simulink model "CryoDetHcd"  (R2016b)
settings: Solver=ode45  StartTime=0.0  StopTime=1e-3  RelTol=1e-3
PreLoadFcn:
  | setup_hcd
values from neighbouring files (symbols this model uses):
  A = sqrt(0.5*erfc(x))    [setup_hcd.m]
  etaRomData = zeros(1,128)    [setup_hcd.m]
  Fadc = 614e6    (= 614000000)    [setup_hcd.m]
  freqRomData = zeros(1,128)    [setup_hcd.m]
  freqRomData1 = zeros(1,128)    [setup_hcd.m]
  freqRomData2 = zeros(1,128)    [setup_hcd.m]
  freqRomData3 = zeros(1,128)    [setup_hcd.m]
undefined symbols (not defined in the file or in its folder): AXI4, B, C, D, j, Lite
libraries: xbsIndex_r4 x2151, CryoDetLibCMB x28, hdlsllib x8, dspsigops x2, simulink x1
(part 13 of 17)

== system CryoDetHcd/DspCore/DSP/channel_processor/channel_processor_x4/128_channel_processor2/Variant Subsystem/LMS/controller/1st_harmonic2 ==
  note: D=16
  note: D=2
  note: D=5
  error : Inport
  gain : Inport  Port=2
  delay : Inport  Port=3
  enable : Inport  Port=4
  cos : Inport  Port=5
  sin : Inport  Port=6
  AddSub4 : xbsIndex_r4/AddSub  mode=Addition  use_carryin=off  use_carryout=off  en=off  latency=3  precision=User Defined  arith_type="Signed  (2's comp)"  n_bits=32  bin_pt=31  quantization=Truncate  overflow=Wrap  use_behavioral_HDL=off  hw_selection=Fabric  pipelined=off  dbl_ovrd=off  block_type=addsub
  Addressable Shift Register : xbsIndex_r4/Addressable Shift Register  infer_latency=off  depth=8  initVector=[0]  en=off  use_behavioral_HDL=off  Optimization=Resource  dbl_ovrd=off  block_type=addrsr
      settings: infoedit="Delay of configurable length.  Any element in the delay line can be addressed and driven onto the output port.<br><br>Hardware notes: Generates fast, compact FIFO-style shift registers or delay lines using SRL16/SRL32 mode of the slice LUTs"
  Addressable Shift Register1 : xbsIndex_r4/Addressable Shift Register  infer_latency=off  depth=8  initVector=[0]  en=off  use_behavioral_HDL=off  Optimization=Resource  dbl_ovrd=off  block_type=addrsr
      settings: infoedit="Delay of configurable length.  Any element in the delay line can be addressed and driven onto the output port.<br><br>Hardware notes: Generates fast, compact FIFO-style shift registers or delay lines using SRL16/SRL32 mode of the slice LUTs"
  Delay1 : xbsIndex_r4/Delay  rst=off  infoeditControl=Selection of Reset will increase slice count due to use of real FFs and instead of SRLs  en=off  latency=5  reg_retiming=off  dbl_ovrd=off  block_type=delay
  Down Sample1 : xbsIndex_r4/Down Sample  sample_ratio=128  sample_phase=First Value of Frame  en=off  rst=off  latency=0  dbl_ovrd=off  block_type=dsamp
  Down Sample2 : xbsIndex_r4/Down Sample  sample_ratio=128  sample_phase=First Value of Frame  en=off  rst=off  latency=0  dbl_ovrd=off  block_type=dsamp
  Down Sample3 : xbsIndex_r4/Down Sample  sample_ratio=128  sample_phase=First Value of Frame  en=off  rst=off  latency=0  dbl_ovrd=off  block_type=dsamp
  Mult{,1,7,13} (4 alike) : xbsIndex_r4/Mult  precision=User Defined  arith_type="Signed  (2's comp)"  n_bits=32  bin_pt=32  quantization=Truncate  overflow=Wrap  en=off  latency=3  use_behavioral_HDL=off  opt=Speed  use_embedded=on  optimum_pipeline=off  pipeline=on  dbl_ovrd=off  use_rpm=on  placement_style=Triangular  block_type=mult
  Subsystem : Subsystem
  Subsystem1 : Subsystem
  Up Sample : xbsIndex_r4/Up Sample  sample_ratio=128  copy_samples=on  en=off  latency=1  dbl_ovrd=off  block_type=usamp
  Up Sample1 : xbsIndex_r4/Up Sample  sample_ratio=128  copy_samples=on  en=off  latency=1  dbl_ovrd=off  block_type=usamp
  interleaved_accumulator1 : Subsystem
  interleaved_accumulator2 : Subsystem
  alpha1 : Outport
  alpha2 : Outport  Port=2
  Out3 : Outport  Port=3
  wires:
  error/1 -> Mult13/1, Mult7/1
  sin/1 -> Down Sample1/1, Mult/2
  cos/1 -> Down Sample2/1, Mult1/2
  Mult7/1 -> Subsystem1/2(in)
  Mult13/1 -> Subsystem/2(in)
  Mult/1 -> AddSub4/1
  Mult1/1 -> AddSub4/2
  AddSub4/1 -> Out3/1
  interleaved_accumulator2/1(Out1) -> alpha2/1, Mult1/1  "alpha2"
  interleaved_accumulator1/1(Out1) -> alpha1/1, Mult/1  "alpha1"
  Subsystem/1(out) -> interleaved_accumulator1/1(In1)
  Down Sample1/1 -> Addressable Shift Register/1
  Down Sample2/1 -> Addressable Shift Register1/1
  Addressable Shift Register1/1 -> Up Sample/1
  Addressable Shift Register/1 -> Up Sample1/1
  delay/1 -> Down Sample3/1
  Subsystem1/1(out) -> interleaved_accumulator2/1(In1)
  gain/1 -> Subsystem1/1(gain), Subsystem/1(gain)
  Down Sample3/1 -> Addressable Shift Register1/2, Addressable Shift Register/2
  Up Sample/1 -> Mult7/2
  Up Sample1/1 -> Mult13/2
  enable/1 -> Delay1/1
  Delay1/1 -> interleaved_accumulator2/2(enable), interleaved_accumulator1/2(enable)

== system CryoDetHcd/DspCore/DSP/channel_processor/channel_processor_x4/128_channel_processor2/Variant Subsystem/LMS/controller/DC ==
  error : Inport
  gain : Inport  Port=2
  dc_offset : Inport  Port=3
  enable : Inport  Port=4
  AddSub4 : xbsIndex_r4/AddSub  mode=Addition  use_carryin=off  use_carryout=off  en=off  latency=3  precision=User Defined  arith_type="Signed  (2's comp)"  n_bits=32  bin_pt=31  quantization=Truncate  overflow=Wrap  use_behavioral_HDL=off  hw_selection=Fabric  pipelined=off  dbl_ovrd=off  block_type=addsub
  Delay : xbsIndex_r4/Delay  rst=off  infoeditControl=Selection of Reset will increase slice count due to use of real FFs and instead of SRLs  en=off  latency=3  reg_retiming=off  dbl_ovrd=off  block_type=delay
  Delay1 : xbsIndex_r4/Delay  rst=off  infoeditControl=Selection of Reset will increase slice count due to use of real FFs and instead of SRLs  en=off  latency=3  reg_retiming=off  dbl_ovrd=off  block_type=delay
  Delay2 : xbsIndex_r4/Delay  rst=off  infoeditControl=Selection of Reset will increase slice count due to use of real FFs and instead of SRLs  en=off  latency=13  reg_retiming=off  dbl_ovrd=off  block_type=delay
  Delay3 : xbsIndex_r4/Delay  rst=off  infoeditControl=Selection of Reset will increase slice count due to use of real FFs and instead of SRLs  en=off  latency=5  reg_retiming=off  dbl_ovrd=off  block_type=delay
  Scope : Scope  NumInputPorts=4
  Subsystem : Subsystem
  interleaved_accumulator2 : Subsystem
  alpha1 : Outport
  Out3 : Outport  Port=2
  wires:
  gain/1 -> Subsystem/1(gain)
  Subsystem/1(out) -> Scope/2, interleaved_accumulator2/1(In1)
  interleaved_accumulator2/1(Out1) -> Scope/3, Delay1/1, alpha1/1  "alpha1"
  AddSub4/1 -> Out3/1
  error/1 -> Scope/1, Delay/1
  dc_offset/1 -> Delay2/1
  Delay/1 -> Subsystem/2(in)
  Delay1/1 -> AddSub4/1
  Delay2/1 -> AddSub4/2
  enable/1 -> Delay3/1
  Delay3/1 -> Scope/4, interleaved_accumulator2/2(enable)

== system CryoDetHcd/DspCore/DSP/channel_processor/channel_processor_x4/128_channel_processor2/Variant Subsystem/LMS/controller/freqs ==
  rst : Inport
  freq : Inport  Port=2
  AddSub : xbsIndex_r4/AddSub  mode=Addition  use_carryin=off  use_carryout=off  en=off  latency=1  precision=User Defined  arith_type=Unsigned  n_bits=16  bin_pt=16  quantization=Truncate  overflow=Wrap  use_behavioral_HDL=off  hw_selection=Fabric  pipelined=off  dbl_ovrd=off  block_type=addsub
  Addressable Shift Register : xbsIndex_r4/Addressable Shift Register  infer_latency=off  depth=128  initVector=[ 1 1 1 zeros(1,125)]  en=off  use_behavioral_HDL=off  Optimization=Resource  dbl_ovrd=off  block_type=addrsr
      settings: infoedit="Delay of configurable length.  Any element in the delay line can be addressed and driven onto the output port.<br><br>Hardware notes: Generates fast, compact FIFO-style shift registers or delay lines using SRL16/SRL32 mode of the slice LUTs"
  Addressable Shift Register1 : xbsIndex_r4/Addressable Shift Register  infer_latency=off  depth=128  initVector=[2 1 0 zeros(1,125)]  en=off  use_behavioral_HDL=off  Optimization=Resource  dbl_ovrd=off  block_type=addrsr
      settings: infoedit="Delay of configurable length.  Any element in the delay line can be addressed and driven onto the output port.<br><br>Hardware notes: Generates fast, compact FIFO-style shift registers or delay lines using SRL16/SRL32 mode of the slice LUTs"
  Assert : xbsIndex_r4/Assert  assert_type=on  type_source=Explicitly  gui_display_data_type=Boolean  arith_type=Boolean  n_bits=16  bin_pt=14  preci_type=Single  exp_width=8  frac_width=24  assert_rate=on  rate_source=Explicitly  period=2/Fadc  output_port=on  block_type=assert
  Assert1 : xbsIndex_r4/Assert  assert_type=on  type_source=Explicitly  gui_display_data_type=Fixed-point  arith_type=Unsigned  n_bits=2  bin_pt=0  preci_type=Single  exp_width=8  frac_width=24  assert_rate=on  rate_source=Explicitly  period=2/Fadc  output_port=on  block_type=assert
  Constant : xbsIndex_r4/Constant  const=126  gui_display_data_type=Fixed-point  arith_type=Unsigned  n_bits=7  bin_pt=0  preci_type=Single  exp_width=8  frac_width=24  explicit_period=off  period=1  equ=P=C  opselect=C  inp2=PCIN>>17  opr=+  inp1=P  carry=CIN  dbl_ovrd=off  block_type=constant
  Constant3 : xbsIndex_r4/Constant  const=126  gui_display_data_type=Fixed-point  arith_type=Unsigned  n_bits=7  bin_pt=0  preci_type=Single  exp_width=8  frac_width=24  explicit_period=off  period=1  equ=P=C  opselect=C  inp2=PCIN>>17  opr=+  inp1=P  carry=CIN  dbl_ovrd=off  block_type=constant
  Constant4 : xbsIndex_r4/Constant  const=1.0  gui_display_data_type=Boolean  arith_type=Boolean  n_bits=16  bin_pt=14  preci_type=Single  exp_width=8  frac_width=24  explicit_period=off  period=1  equ=P=C  opselect=C  inp2=PCIN>>17  opr=+  inp1=P  carry=CIN  dbl_ovrd=off  block_type=constant
  Constant5 : xbsIndex_r4/Constant  const=0  gui_display_data_type=Boolean  arith_type=Boolean  n_bits=16  bin_pt=14  preci_type=Single  exp_width=8  frac_width=24  explicit_period=off  period=1  equ=P=C  opselect=C  inp2=PCIN>>17  opr=+  inp1=P  carry=CIN  dbl_ovrd=off  block_type=constant
  Constant6 : xbsIndex_r4/Constant  const=0  gui_display_data_type=Fixed-point  arith_type=Unsigned  n_bits=2  bin_pt=0  preci_type=Single  exp_width=8  frac_width=24  explicit_period=off  period=1  equ=P=C  opselect=C  inp2=PCIN>>17  opr=+  inp1=P  carry=CIN  dbl_ovrd=off  block_type=constant
  Constant7 : xbsIndex_r4/Constant  const=1  gui_display_data_type=Fixed-point  arith_type=Unsigned  n_bits=2  bin_pt=0  preci_type=Single  exp_width=8  frac_width=24  explicit_period=off  period=1  equ=P=C  opselect=C  inp2=PCIN>>17  opr=+  inp1=P  carry=CIN  dbl_ovrd=off  block_type=constant
  Constant8 : xbsIndex_r4/Constant  const=2  gui_display_data_type=Fixed-point  arith_type=Unsigned  n_bits=2  bin_pt=0  preci_type=Single  exp_width=8  frac_width=24  explicit_period=off  period=1  equ=P=C  opselect=C  inp2=PCIN>>17  opr=+  inp1=P  carry=CIN  dbl_ovrd=off  block_type=constant
  "DDS Compiler 6.0 " : xbsIndex_r4/DDS Compiler 6.0   partspresent=Phase_Generator_and_SIN_COS_LUT  dds_clock_rate=38.4  channels=3  mode_of_operation=Standard  modulus=9  parameter_entry=Hardware_Parameters  spurious_free_dynamic_range=45  frequency_resolution=0.4  noise_shaping=None  phase_width=16  output_width=18  output_selection=Sine_and_Cosine  negative_sine=off  negative_cosine=off  amplitude_mode=Full_Range  memory_type=Auto  optimization_goal=Speed  dsp48_use=Minimal  resync=off  latency_configuration=Auto  latency=1  has_phase_out=off  has_aclken=off  has_aresetn=on  explicit_period=off  period=1  data_has_tlast=Not_Required  has_tready=on  s_phase_has_tuser=User_Field  m_data_has_tuser=User_Field  m_phase_has_tuser=Not_Required  s_phase_tuser_width=2  output_form=Twos_Complement  s_config_sync_mode=On_Packet  phase_increment=Streaming  output_frequency1=0  output_frequency2=0  output_frequency3=0  output_frequency4=0  output_frequency5=0  output_frequency6=0  output_frequency7=0  output_frequency8=0  output_frequency9=0  output_frequency10=0  output_frequency11=0  output_frequency12=0  output_frequency13=0  output_frequency14=0  output_frequency15=0  output_frequency16=0  pinc1='0'  pinc2='0'  pinc3='0'  pinc4='0'  pinc5='0'  pinc6='0'  pinc7='0'  pinc8='0'  pinc9='0'  pinc10='0'  pinc11='0'  pinc12='0'  pinc13='0'  pinc14='0'  pinc15='0'  pinc16='0'  phase_offset=None  phase_offset_angles1=0  phase_offset_angles2=0  phase_offset_angles3=0  phase_offset_angles4=0  phase_offset_angles5=0  phase_offset_angles6=0  phase_offset_angles7=0  phase_offset_angles8=0  phase_offset_angles9=0  phase_offset_angles10=0  phase_offset_angles11=0  phase_offset_angles12=0  phase_offset_angles13=0  phase_offset_angles14=0  phase_offset_angles15=0  phase_offset_angles16=0  poff1='0'  poff2='0'  poff3='0'  poff4='0'  poff5='0'  poff6='0'  poff7='0'  poff8='0'  poff9='0'  poff10='0'  poff11='0'  poff12='0'  poff13='0'  poff14='0'  poff15='0'  poff16='0'  trim_axipin_name=on  simulation_type=hybrid_sim  simulation_model=sysgen:xddsv6_0_cmodel  data_path_portlist={ 's_axis_config_tdata_poff', 's_axis_config_tdata_chan0_poff', 's_axis_config_tdata_pinc', 's_axis_config_tdata_chan0_pinc', 's_axis_phase_tdata_resync', 's_axis_phase_tdata_chan0_resync', 's_axis_phase_tdata_poff', 's_axis_phase_tdata_chan0_poff', 's_axis_phase_tdata_pinc', 's_axis_phase_tdata_chan0_pinc', 's_axis_phase_tdata_phase_in', 'm_axis_data_tdata_sine', 'm_axis_data_tdata_chan0_sine', 'm_axis_data_tdata_cosine', 'm_axis_data_tdata_chan0_cosine', 'm_axis_phase_tdata_phase_out', 'm_axis_phase_tdata_chan0_phase_out'}  por_mode=false  gui_behaviour=Sysgen  ip_name=DDS Compiler  ip_version=6.0  dsptool_ready=true  wrapper_available=true  port_translation_map={ 'aclken' => 'en', 'aresetn' => 'rst' }  ipcore_usecache=true  ipcore_useipmodelcache=true  ipcore_xco_need_fpga_part=true  ipcore_verbose=false  block_type=dds_compiler_v6_0
  Inverter : xbsIndex_r4/Inverter  en=off  latency=0  dbl_ovrd=off  block_type=inv
  Mux5 : xbsIndex_r4/Mux  inputs=3  en=off  latency=1  precision=Full  arith_type=Unsigned  n_bits=16  bin_pt=14  quantization=Truncate  overflow=Wrap  dbl_ovrd=off  block_type=mux
  Register{1..3,8,12..16} (9 alike) : xbsIndex_r4/Register  init=0  rst=off  en=off  dbl_ovrd=off  block_type=register
  Shift : xbsIndex_r4/Shift  shift_dir=Left  shift_bits=1  en=off  latency=1  precision=User Defined  arith_type=Unsigned  n_bits=16  bin_pt=16  quantization=Truncate  overflow=Wrap  dbl_ovrd=off  block_type=shift
  Subsystem : Subsystem
  Subsystem1 : Subsystem
  Subsystem2 : Subsystem
  Terminator : Terminator
  Terminator1 : Terminator
  Terminator2 : Terminator
  h0_0 : Outport
  h0_1 : Outport  Port=2
  h1_0 : Outport  Port=3
  h1_1 : Outport  Port=4
  h2_0 : Outport  Port=5
  h2_1 : Outport  Port=6
  wires:
  "DDS Compiler 6.0 "/7 -> Terminator2/1
  "DDS Compiler 6.0 "/1 -> Terminator/1
  "DDS Compiler 6.0 "/6 -> Terminator1/1
  Addressable Shift Register/1 -> Register8/1
  Register8/1 -> Register13/1, Assert/1
  Constant/1 -> Addressable Shift Register/2
  Addressable Shift Register1/1 -> Register12/1
  Register12/1 -> Register1/1, Mux5/1, Assert1/1
  Constant3/1 -> Addressable Shift Register1/2
  Register13/1 -> "DDS Compiler 6.0 "/1
  Register14/1 -> Shift/1, AddSub/1, Mux5/2
  Shift/1 -> AddSub/2, Mux5/3
  AddSub/1 -> Mux5/4
  Mux5/1 -> "DDS Compiler 6.0 "/2
  Constant4/1 -> "DDS Compiler 6.0 "/5
  Constant5/1 -> "DDS Compiler 6.0 "/3
  "DDS Compiler 6.0 "/2 -> Register2/1
  "DDS Compiler 6.0 "/3 -> Register15/1
  "DDS Compiler 6.0 "/4 -> Register16/1
  Register15/1 -> Subsystem/3(In3), Subsystem2/3(In3), Subsystem1/3(In3)
  Constant6/1 -> Subsystem/1(Chan)
  Constant8/1 -> Subsystem2/1(Chan)
  Constant7/1 -> Subsystem1/1(Chan)
  freq/1 -> Register14/1
  Assert/1 -> Addressable Shift Register/1
  Assert1/1 -> Addressable Shift Register1/1
  Register3/1 -> Subsystem/2(In2), Subsystem2/2(In2), Subsystem1/2(In2)
  Register2/1 -> Subsystem2/5(valid), Subsystem1/5(valid), Subsystem/5(valid)
  Register16/1 -> Subsystem1/4(In4), Subsystem/4(In4), Subsystem2/4(In4)
  rst/1 -> Inverter/1
  Inverter/1 -> "DDS Compiler 6.0 "/6
  Register1/1 -> "DDS Compiler 6.0 "/4
  "DDS Compiler 6.0 "/5 -> Register3/1
  Subsystem2/2(Out3) -> h2_1/1
  Subsystem2/1(Out2) -> h2_0/1
  Subsystem1/2(Out3) -> h1_1/1
  Subsystem1/1(Out2) -> h1_0/1
  Subsystem/2(Out3) -> h0_1/1
  Subsystem/1(Out2) -> h0_0/1

== system CryoDetHcd/DspCore/DSP/channel_processor/channel_processor_x4/128_channel_processor3/Variant Subsystem/LMS/controller/1st_harmonic ==
  note: D=5
  note: D=2
  note: D=16
  error : Inport
  gain : Inport  Port=2
  delay : Inport  Port=3
  enable : Inport  Port=4
  cos : Inport  Port=5
  sin : Inport  Port=6
  AddSub4 : xbsIndex_r4/AddSub  mode=Addition  use_carryin=off  use_carryout=off  en=off  latency=3  precision=User Defined  arith_type="Signed  (2's comp)"  n_bits=32  bin_pt=31  quantization=Truncate  overflow=Wrap  use_behavioral_HDL=off  hw_selection=Fabric  pipelined=off  dbl_ovrd=off  block_type=addsub
  Addressable Shift Register : xbsIndex_r4/Addressable Shift Register  infer_latency=off  depth=8  initVector=[0]  en=off  use_behavioral_HDL=off  Optimization=Resource  dbl_ovrd=off  block_type=addrsr
      settings: infoedit="Delay of configurable length.  Any element in the delay line can be addressed and driven onto the output port.<br><br>Hardware notes: Generates fast, compact FIFO-style shift registers or delay lines using SRL16/SRL32 mode of the slice LUTs"
  Addressable Shift Register1 : xbsIndex_r4/Addressable Shift Register  infer_latency=off  depth=8  initVector=[0]  en=off  use_behavioral_HDL=off  Optimization=Resource  dbl_ovrd=off  block_type=addrsr
      settings: infoedit="Delay of configurable length.  Any element in the delay line can be addressed and driven onto the output port.<br><br>Hardware notes: Generates fast, compact FIFO-style shift registers or delay lines using SRL16/SRL32 mode of the slice LUTs"
  Delay1 : xbsIndex_r4/Delay  rst=off  infoeditControl=Selection of Reset will increase slice count due to use of real FFs and instead of SRLs  en=off  latency=5  reg_retiming=off  dbl_ovrd=off  block_type=delay
  Down Sample1 : xbsIndex_r4/Down Sample  sample_ratio=128  sample_phase=First Value of Frame  en=off  rst=off  latency=0  dbl_ovrd=off  block_type=dsamp
  Down Sample2 : xbsIndex_r4/Down Sample  sample_ratio=128  sample_phase=First Value of Frame  en=off  rst=off  latency=0  dbl_ovrd=off  block_type=dsamp
  Down Sample3 : xbsIndex_r4/Down Sample  sample_ratio=128  sample_phase=First Value of Frame  en=off  rst=off  latency=0  dbl_ovrd=off  block_type=dsamp
  Mult{,1,7,13} (4 alike) : xbsIndex_r4/Mult  precision=User Defined  arith_type="Signed  (2's comp)"  n_bits=32  bin_pt=32  quantization=Truncate  overflow=Wrap  en=off  latency=3  use_behavioral_HDL=off  opt=Speed  use_embedded=on  optimum_pipeline=off  pipeline=on  dbl_ovrd=off  use_rpm=on  placement_style=Triangular  block_type=mult
  Subsystem : Subsystem
  Subsystem1 : Subsystem
  Up Sample : xbsIndex_r4/Up Sample  sample_ratio=128  copy_samples=on  en=off  latency=1  dbl_ovrd=off  block_type=usamp
  Up Sample1 : xbsIndex_r4/Up Sample  sample_ratio=128  copy_samples=on  en=off  latency=1  dbl_ovrd=off  block_type=usamp
  interleaved_accumulator1 : Subsystem
  interleaved_accumulator2 : Subsystem
  alpha1 : Outport
  alpha2 : Outport  Port=2
  Out3 : Outport  Port=3
  wires:
  Delay1/1 -> interleaved_accumulator1/2(enable), interleaved_accumulator2/2(enable)
  enable/1 -> Delay1/1
  Up Sample1/1 -> Mult13/2
  Up Sample/1 -> Mult7/2
  Down Sample3/1 -> Addressable Shift Register/2, Addressable Shift Register1/2
  gain/1 -> Subsystem/1(gain), Subsystem1/1(gain)
  Subsystem1/1(out) -> interleaved_accumulator2/1(In1)
  delay/1 -> Down Sample3/1
  Addressable Shift Register/1 -> Up Sample1/1
  Addressable Shift Register1/1 -> Up Sample/1
  Down Sample2/1 -> Addressable Shift Register1/1
  Down Sample1/1 -> Addressable Shift Register/1
  Subsystem/1(out) -> interleaved_accumulator1/1(In1)
  interleaved_accumulator1/1(Out1) -> Mult/1, alpha1/1  "alpha1"
  interleaved_accumulator2/1(Out1) -> Mult1/1, alpha2/1  "alpha2"
  AddSub4/1 -> Out3/1
  Mult1/1 -> AddSub4/2
  Mult/1 -> AddSub4/1
  Mult13/1 -> Subsystem/2(in)
  Mult7/1 -> Subsystem1/2(in)
  cos/1 -> Mult1/2, Down Sample2/1
  sin/1 -> Mult/2, Down Sample1/1
  error/1 -> Mult7/1, Mult13/1

== system CryoDetHcd/DspCore/DSP/channel_processor/channel_processor_x4/128_channel_processor3/Variant Subsystem/LMS/controller/1st_harmonic1 ==
  note: D=16
  note: D=2
  note: D=5
  error : Inport
  gain : Inport  Port=2
  delay : Inport  Port=3
  enable : Inport  Port=4
  cos : Inport  Port=5
  sin : Inport  Port=6
  AddSub4 : xbsIndex_r4/AddSub  mode=Addition  use_carryin=off  use_carryout=off  en=off  latency=3  precision=User Defined  arith_type="Signed  (2's comp)"  n_bits=32  bin_pt=31  quantization=Truncate  overflow=Wrap  use_behavioral_HDL=off  hw_selection=Fabric  pipelined=off  dbl_ovrd=off  block_type=addsub
  Addressable Shift Register : xbsIndex_r4/Addressable Shift Register  infer_latency=off  depth=8  initVector=[0]  en=off  use_behavioral_HDL=off  Optimization=Resource  dbl_ovrd=off  block_type=addrsr
      settings: infoedit="Delay of configurable length.  Any element in the delay line can be addressed and driven onto the output port.<br><br>Hardware notes: Generates fast, compact FIFO-style shift registers or delay lines using SRL16/SRL32 mode of the slice LUTs"
  Addressable Shift Register1 : xbsIndex_r4/Addressable Shift Register  infer_latency=off  depth=8  initVector=[0]  en=off  use_behavioral_HDL=off  Optimization=Resource  dbl_ovrd=off  block_type=addrsr
      settings: infoedit="Delay of configurable length.  Any element in the delay line can be addressed and driven onto the output port.<br><br>Hardware notes: Generates fast, compact FIFO-style shift registers or delay lines using SRL16/SRL32 mode of the slice LUTs"
  Delay1 : xbsIndex_r4/Delay  rst=off  infoeditControl=Selection of Reset will increase slice count due to use of real FFs and instead of SRLs  en=off  latency=5  reg_retiming=off  dbl_ovrd=off  block_type=delay
  Down Sample1 : xbsIndex_r4/Down Sample  sample_ratio=128  sample_phase=First Value of Frame  en=off  rst=off  latency=0  dbl_ovrd=off  block_type=dsamp
  Down Sample2 : xbsIndex_r4/Down Sample  sample_ratio=128  sample_phase=First Value of Frame  en=off  rst=off  latency=0  dbl_ovrd=off  block_type=dsamp
  Down Sample3 : xbsIndex_r4/Down Sample  sample_ratio=128  sample_phase=First Value of Frame  en=off  rst=off  latency=0  dbl_ovrd=off  block_type=dsamp
  Mult{,1,7,13} (4 alike) : xbsIndex_r4/Mult  precision=User Defined  arith_type="Signed  (2's comp)"  n_bits=32  bin_pt=32  quantization=Truncate  overflow=Wrap  en=off  latency=3  use_behavioral_HDL=off  opt=Speed  use_embedded=on  optimum_pipeline=off  pipeline=on  dbl_ovrd=off  use_rpm=on  placement_style=Triangular  block_type=mult
  Subsystem : Subsystem
  Subsystem1 : Subsystem
  Up Sample : xbsIndex_r4/Up Sample  sample_ratio=128  copy_samples=on  en=off  latency=1  dbl_ovrd=off  block_type=usamp
  Up Sample1 : xbsIndex_r4/Up Sample  sample_ratio=128  copy_samples=on  en=off  latency=1  dbl_ovrd=off  block_type=usamp
  interleaved_accumulator1 : Subsystem
  interleaved_accumulator2 : Subsystem
  alpha1 : Outport
  alpha2 : Outport  Port=2
  Out3 : Outport  Port=3
  wires:
  error/1 -> Mult13/1, Mult7/1
  sin/1 -> Down Sample1/1, Mult/2
  cos/1 -> Down Sample2/1, Mult1/2
  Mult7/1 -> Subsystem1/2(in)
  Mult13/1 -> Subsystem/2(in)
  Mult/1 -> AddSub4/1
  Mult1/1 -> AddSub4/2
  AddSub4/1 -> Out3/1
  interleaved_accumulator2/1(Out1) -> alpha2/1, Mult1/1  "alpha2"
  interleaved_accumulator1/1(Out1) -> alpha1/1, Mult/1  "alpha1"
  Subsystem/1(out) -> interleaved_accumulator1/1(In1)
  Down Sample1/1 -> Addressable Shift Register/1
  Down Sample2/1 -> Addressable Shift Register1/1
  Addressable Shift Register1/1 -> Up Sample/1
  Addressable Shift Register/1 -> Up Sample1/1
  delay/1 -> Down Sample3/1
  Subsystem1/1(out) -> interleaved_accumulator2/1(In1)
  gain/1 -> Subsystem1/1(gain), Subsystem/1(gain)
  Down Sample3/1 -> Addressable Shift Register1/2, Addressable Shift Register/2
  Up Sample/1 -> Mult7/2
  Up Sample1/1 -> Mult13/2
  enable/1 -> Delay1/1
  Delay1/1 -> interleaved_accumulator2/2(enable), interleaved_accumulator1/2(enable)

== system CryoDetHcd/DspCore/DSP/channel_processor/channel_processor_x4/128_channel_processor3/Variant Subsystem/LMS/controller/1st_harmonic2 ==
  note: D=5
  note: D=2
  note: D=16
  error : Inport
  gain : Inport  Port=2
  delay : Inport  Port=3
  enable : Inport  Port=4
  cos : Inport  Port=5
  sin : Inport  Port=6
  AddSub4 : xbsIndex_r4/AddSub  mode=Addition  use_carryin=off  use_carryout=off  en=off  latency=3  precision=User Defined  arith_type="Signed  (2's comp)"  n_bits=32  bin_pt=31  quantization=Truncate  overflow=Wrap  use_behavioral_HDL=off  hw_selection=Fabric  pipelined=off  dbl_ovrd=off  block_type=addsub
  Addressable Shift Register : xbsIndex_r4/Addressable Shift Register  infer_latency=off  depth=8  initVector=[0]  en=off  use_behavioral_HDL=off  Optimization=Resource  dbl_ovrd=off  block_type=addrsr
      settings: infoedit="Delay of configurable length.  Any element in the delay line can be addressed and driven onto the output port.<br><br>Hardware notes: Generates fast, compact FIFO-style shift registers or delay lines using SRL16/SRL32 mode of the slice LUTs"
  Addressable Shift Register1 : xbsIndex_r4/Addressable Shift Register  infer_latency=off  depth=8  initVector=[0]  en=off  use_behavioral_HDL=off  Optimization=Resource  dbl_ovrd=off  block_type=addrsr
      settings: infoedit="Delay of configurable length.  Any element in the delay line can be addressed and driven onto the output port.<br><br>Hardware notes: Generates fast, compact FIFO-style shift registers or delay lines using SRL16/SRL32 mode of the slice LUTs"
  Delay1 : xbsIndex_r4/Delay  rst=off  infoeditControl=Selection of Reset will increase slice count due to use of real FFs and instead of SRLs  en=off  latency=5  reg_retiming=off  dbl_ovrd=off  block_type=delay
  Down Sample1 : xbsIndex_r4/Down Sample  sample_ratio=128  sample_phase=First Value of Frame  en=off  rst=off  latency=0  dbl_ovrd=off  block_type=dsamp
  Down Sample2 : xbsIndex_r4/Down Sample  sample_ratio=128  sample_phase=First Value of Frame  en=off  rst=off  latency=0  dbl_ovrd=off  block_type=dsamp
  Down Sample3 : xbsIndex_r4/Down Sample  sample_ratio=128  sample_phase=First Value of Frame  en=off  rst=off  latency=0  dbl_ovrd=off  block_type=dsamp
  Mult{,1,7,13} (4 alike) : xbsIndex_r4/Mult  precision=User Defined  arith_type="Signed  (2's comp)"  n_bits=32  bin_pt=32  quantization=Truncate  overflow=Wrap  en=off  latency=3  use_behavioral_HDL=off  opt=Speed  use_embedded=on  optimum_pipeline=off  pipeline=on  dbl_ovrd=off  use_rpm=on  placement_style=Triangular  block_type=mult
  Subsystem : Subsystem
  Subsystem1 : Subsystem
  Up Sample : xbsIndex_r4/Up Sample  sample_ratio=128  copy_samples=on  en=off  latency=1  dbl_ovrd=off  block_type=usamp
  Up Sample1 : xbsIndex_r4/Up Sample  sample_ratio=128  copy_samples=on  en=off  latency=1  dbl_ovrd=off  block_type=usamp
  interleaved_accumulator1 : Subsystem
  interleaved_accumulator2 : Subsystem
  alpha1 : Outport
  alpha2 : Outport  Port=2
  Out3 : Outport  Port=3
  wires:
  Delay1/1 -> interleaved_accumulator1/2(enable), interleaved_accumulator2/2(enable)
  enable/1 -> Delay1/1
  Up Sample1/1 -> Mult13/2
  Up Sample/1 -> Mult7/2
  Down Sample3/1 -> Addressable Shift Register/2, Addressable Shift Register1/2
  gain/1 -> Subsystem/1(gain), Subsystem1/1(gain)
  Subsystem1/1(out) -> interleaved_accumulator2/1(In1)
  delay/1 -> Down Sample3/1
  Addressable Shift Register/1 -> Up Sample1/1
  Addressable Shift Register1/1 -> Up Sample/1
  Down Sample2/1 -> Addressable Shift Register1/1
  Down Sample1/1 -> Addressable Shift Register/1
  Subsystem/1(out) -> interleaved_accumulator1/1(In1)
  interleaved_accumulator1/1(Out1) -> Mult/1, alpha1/1  "alpha1"
  interleaved_accumulator2/1(Out1) -> Mult1/1, alpha2/1  "alpha2"
  AddSub4/1 -> Out3/1
  Mult1/1 -> AddSub4/2
  Mult/1 -> AddSub4/1
  Mult13/1 -> Subsystem/2(in)
  Mult7/1 -> Subsystem1/2(in)
  cos/1 -> Mult1/2, Down Sample2/1
  sin/1 -> Mult/2, Down Sample1/1
  error/1 -> Mult7/1, Mult13/1

== system CryoDetHcd/DspCore/DSP/channel_processor/channel_processor_x4/128_channel_processor3/Variant Subsystem/LMS/controller/DC ==
  error : Inport
  gain : Inport  Port=2
  dc_offset : Inport  Port=3
  enable : Inport  Port=4
  AddSub4 : xbsIndex_r4/AddSub  mode=Addition  use_carryin=off  use_carryout=off  en=off  latency=3  precision=User Defined  arith_type="Signed  (2's comp)"  n_bits=32  bin_pt=31  quantization=Truncate  overflow=Wrap  use_behavioral_HDL=off  hw_selection=Fabric  pipelined=off  dbl_ovrd=off  block_type=addsub
  Delay : xbsIndex_r4/Delay  rst=off  infoeditControl=Selection of Reset will increase slice count due to use of real FFs and instead of SRLs  en=off  latency=3  reg_retiming=off  dbl_ovrd=off  block_type=delay
  Delay1 : xbsIndex_r4/Delay  rst=off  infoeditControl=Selection of Reset will increase slice count due to use of real FFs and instead of SRLs  en=off  latency=3  reg_retiming=off  dbl_ovrd=off  block_type=delay
  Delay2 : xbsIndex_r4/Delay  rst=off  infoeditControl=Selection of Reset will increase slice count due to use of real FFs and instead of SRLs  en=off  latency=13  reg_retiming=off  dbl_ovrd=off  block_type=delay
  Delay3 : xbsIndex_r4/Delay  rst=off  infoeditControl=Selection of Reset will increase slice count due to use of real FFs and instead of SRLs  en=off  latency=5  reg_retiming=off  dbl_ovrd=off  block_type=delay
  Scope : Scope  NumInputPorts=4
  Subsystem : Subsystem
  interleaved_accumulator2 : Subsystem
  alpha1 : Outport
  Out3 : Outport  Port=2
  wires:
  Delay3/1 -> interleaved_accumulator2/2(enable), Scope/4
  enable/1 -> Delay3/1
  Delay2/1 -> AddSub4/2
  Delay1/1 -> AddSub4/1
  Delay/1 -> Subsystem/2(in)
  dc_offset/1 -> Delay2/1
  error/1 -> Delay/1, Scope/1
  AddSub4/1 -> Out3/1
  interleaved_accumulator2/1(Out1) -> alpha1/1, Delay1/1, Scope/3  "alpha1"
  Subsystem/1(out) -> interleaved_accumulator2/1(In1), Scope/2
  gain/1 -> Subsystem/1(gain)

== system CryoDetHcd/DspCore/DSP/channel_processor/channel_processor_x4/128_channel_processor3/Variant Subsystem/LMS/controller/freqs ==
  rst : Inport
  freq : Inport  Port=2
  AddSub : xbsIndex_r4/AddSub  mode=Addition  use_carryin=off  use_carryout=off  en=off  latency=1  precision=User Defined  arith_type=Unsigned  n_bits=16  bin_pt=16  quantization=Truncate  overflow=Wrap  use_behavioral_HDL=off  hw_selection=Fabric  pipelined=off  dbl_ovrd=off  block_type=addsub
  Addressable Shift Register : xbsIndex_r4/Addressable Shift Register  infer_latency=off  depth=128  initVector=[ 1 1 1 zeros(1,125)]  en=off  use_behavioral_HDL=off  Optimization=Resource  dbl_ovrd=off  block_type=addrsr
      settings: infoedit="Delay of configurable length.  Any element in the delay line can be addressed and driven onto the output port.<br><br>Hardware notes: Generates fast, compact FIFO-style shift registers or delay lines using SRL16/SRL32 mode of the slice LUTs"
  Addressable Shift Register1 : xbsIndex_r4/Addressable Shift Register  infer_latency=off  depth=128  initVector=[2 1 0 zeros(1,125)]  en=off  use_behavioral_HDL=off  Optimization=Resource  dbl_ovrd=off  block_type=addrsr
      settings: infoedit="Delay of configurable length.  Any element in the delay line can be addressed and driven onto the output port.<br><br>Hardware notes: Generates fast, compact FIFO-style shift registers or delay lines using SRL16/SRL32 mode of the slice LUTs"
  Assert : xbsIndex_r4/Assert  assert_type=on  type_source=Explicitly  gui_display_data_type=Boolean  arith_type=Boolean  n_bits=16  bin_pt=14  preci_type=Single  exp_width=8  frac_width=24  assert_rate=on  rate_source=Explicitly  period=2/Fadc  output_port=on  block_type=assert
  Assert1 : xbsIndex_r4/Assert  assert_type=on  type_source=Explicitly  gui_display_data_type=Fixed-point  arith_type=Unsigned  n_bits=2  bin_pt=0  preci_type=Single  exp_width=8  frac_width=24  assert_rate=on  rate_source=Explicitly  period=2/Fadc  output_port=on  block_type=assert
  Constant : xbsIndex_r4/Constant  const=126  gui_display_data_type=Fixed-point  arith_type=Unsigned  n_bits=7  bin_pt=0  preci_type=Single  exp_width=8  frac_width=24  explicit_period=off  period=1  equ=P=C  opselect=C  inp2=PCIN>>17  opr=+  inp1=P  carry=CIN  dbl_ovrd=off  block_type=constant
  Constant3 : xbsIndex_r4/Constant  const=126  gui_display_data_type=Fixed-point  arith_type=Unsigned  n_bits=7  bin_pt=0  preci_type=Single  exp_width=8  frac_width=24  explicit_period=off  period=1  equ=P=C  opselect=C  inp2=PCIN>>17  opr=+  inp1=P  carry=CIN  dbl_ovrd=off  block_type=constant
  Constant4 : xbsIndex_r4/Constant  const=1.0  gui_display_data_type=Boolean  arith_type=Boolean  n_bits=16  bin_pt=14  preci_type=Single  exp_width=8  frac_width=24  explicit_period=off  period=1  equ=P=C  opselect=C  inp2=PCIN>>17  opr=+  inp1=P  carry=CIN  dbl_ovrd=off  block_type=constant
  Constant5 : xbsIndex_r4/Constant  const=0  gui_display_data_type=Boolean  arith_type=Boolean  n_bits=16  bin_pt=14  preci_type=Single  exp_width=8  frac_width=24  explicit_period=off  period=1  equ=P=C  opselect=C  inp2=PCIN>>17  opr=+  inp1=P  carry=CIN  dbl_ovrd=off  block_type=constant
  Constant6 : xbsIndex_r4/Constant  const=0  gui_display_data_type=Fixed-point  arith_type=Unsigned  n_bits=2  bin_pt=0  preci_type=Single  exp_width=8  frac_width=24  explicit_period=off  period=1  equ=P=C  opselect=C  inp2=PCIN>>17  opr=+  inp1=P  carry=CIN  dbl_ovrd=off  block_type=constant
  Constant7 : xbsIndex_r4/Constant  const=1  gui_display_data_type=Fixed-point  arith_type=Unsigned  n_bits=2  bin_pt=0  preci_type=Single  exp_width=8  frac_width=24  explicit_period=off  period=1  equ=P=C  opselect=C  inp2=PCIN>>17  opr=+  inp1=P  carry=CIN  dbl_ovrd=off  block_type=constant
  Constant8 : xbsIndex_r4/Constant  const=2  gui_display_data_type=Fixed-point  arith_type=Unsigned  n_bits=2  bin_pt=0  preci_type=Single  exp_width=8  frac_width=24  explicit_period=off  period=1  equ=P=C  opselect=C  inp2=PCIN>>17  opr=+  inp1=P  carry=CIN  dbl_ovrd=off  block_type=constant
  "DDS Compiler 6.0 " : xbsIndex_r4/DDS Compiler 6.0   partspresent=Phase_Generator_and_SIN_COS_LUT  dds_clock_rate=38.4  channels=3  mode_of_operation=Standard  modulus=9  parameter_entry=Hardware_Parameters  spurious_free_dynamic_range=45  frequency_resolution=0.4  noise_shaping=None  phase_width=16  output_width=18  output_selection=Sine_and_Cosine  negative_sine=off  negative_cosine=off  amplitude_mode=Full_Range  memory_type=Auto  optimization_goal=Speed  dsp48_use=Minimal  resync=off  latency_configuration=Auto  latency=1  has_phase_out=off  has_aclken=off  has_aresetn=on  explicit_period=off  period=1  data_has_tlast=Not_Required  has_tready=on  s_phase_has_tuser=User_Field  m_data_has_tuser=User_Field  m_phase_has_tuser=Not_Required  s_phase_tuser_width=2  output_form=Twos_Complement  s_config_sync_mode=On_Packet  phase_increment=Streaming  output_frequency1=0  output_frequency2=0  output_frequency3=0  output_frequency4=0  output_frequency5=0  output_frequency6=0  output_frequency7=0  output_frequency8=0  output_frequency9=0  output_frequency10=0  output_frequency11=0  output_frequency12=0  output_frequency13=0  output_frequency14=0  output_frequency15=0  output_frequency16=0  pinc1='0'  pinc2='0'  pinc3='0'  pinc4='0'  pinc5='0'  pinc6='0'  pinc7='0'  pinc8='0'  pinc9='0'  pinc10='0'  pinc11='0'  pinc12='0'  pinc13='0'  pinc14='0'  pinc15='0'  pinc16='0'  phase_offset=None  phase_offset_angles1=0  phase_offset_angles2=0  phase_offset_angles3=0  phase_offset_angles4=0  phase_offset_angles5=0  phase_offset_angles6=0  phase_offset_angles7=0  phase_offset_angles8=0  phase_offset_angles9=0  phase_offset_angles10=0  phase_offset_angles11=0  phase_offset_angles12=0  phase_offset_angles13=0  phase_offset_angles14=0  phase_offset_angles15=0  phase_offset_angles16=0  poff1='0'  poff2='0'  poff3='0'  poff4='0'  poff5='0'  poff6='0'  poff7='0'  poff8='0'  poff9='0'  poff10='0'  poff11='0'  poff12='0'  poff13='0'  poff14='0'  poff15='0'  poff16='0'  trim_axipin_name=on  simulation_type=hybrid_sim  simulation_model=sysgen:xddsv6_0_cmodel  data_path_portlist={ 's_axis_config_tdata_poff', 's_axis_config_tdata_chan0_poff', 's_axis_config_tdata_pinc', 's_axis_config_tdata_chan0_pinc', 's_axis_phase_tdata_resync', 's_axis_phase_tdata_chan0_resync', 's_axis_phase_tdata_poff', 's_axis_phase_tdata_chan0_poff', 's_axis_phase_tdata_pinc', 's_axis_phase_tdata_chan0_pinc', 's_axis_phase_tdata_phase_in', 'm_axis_data_tdata_sine', 'm_axis_data_tdata_chan0_sine', 'm_axis_data_tdata_cosine', 'm_axis_data_tdata_chan0_cosine', 'm_axis_phase_tdata_phase_out', 'm_axis_phase_tdata_chan0_phase_out'}  por_mode=false  gui_behaviour=Sysgen  ip_name=DDS Compiler  ip_version=6.0  dsptool_ready=true  wrapper_available=true  port_translation_map={ 'aclken' => 'en', 'aresetn' => 'rst' }  ipcore_usecache=true  ipcore_useipmodelcache=true  ipcore_xco_need_fpga_part=true  ipcore_verbose=false  block_type=dds_compiler_v6_0
  Inverter : xbsIndex_r4/Inverter  en=off  latency=0  dbl_ovrd=off  block_type=inv
  Mux5 : xbsIndex_r4/Mux  inputs=3  en=off  latency=1  precision=Full  arith_type=Unsigned  n_bits=16  bin_pt=14  quantization=Truncate  overflow=Wrap  dbl_ovrd=off  block_type=mux
  Register{1..3,8,12..16} (9 alike) : xbsIndex_r4/Register  init=0  rst=off  en=off  dbl_ovrd=off  block_type=register
  Shift : xbsIndex_r4/Shift  shift_dir=Left  shift_bits=1  en=off  latency=1  precision=User Defined  arith_type=Unsigned  n_bits=16  bin_pt=16  quantization=Truncate  overflow=Wrap  dbl_ovrd=off  block_type=shift
  Subsystem : Subsystem
  Subsystem1 : Subsystem
  Subsystem2 : Subsystem
  Terminator : Terminator
  Terminator1 : Terminator
  Terminator2 : Terminator
  h0_0 : Outport
  h0_1 : Outport  Port=2
  h1_0 : Outport  Port=3
  h1_1 : Outport  Port=4
  h2_0 : Outport  Port=5
  h2_1 : Outport  Port=6
  wires:
  Subsystem/1(Out2) -> h0_0/1
  Subsystem/2(Out3) -> h0_1/1
  Subsystem1/1(Out2) -> h1_0/1
  Subsystem1/2(Out3) -> h1_1/1
  Subsystem2/1(Out2) -> h2_0/1
  Subsystem2/2(Out3) -> h2_1/1
  "DDS Compiler 6.0 "/5 -> Register3/1
  Register1/1 -> "DDS Compiler 6.0 "/4
  Inverter/1 -> "DDS Compiler 6.0 "/6
  rst/1 -> Inverter/1
  Register16/1 -> Subsystem2/4(In4), Subsystem/4(In4), Subsystem1/4(In4)
  Register2/1 -> Subsystem/5(valid), Subsystem1/5(valid), Subsystem2/5(valid)
  Register3/1 -> Subsystem1/2(In2), Subsystem2/2(In2), Subsystem/2(In2)
  Assert1/1 -> Addressable Shift Register1/1
  Assert/1 -> Addressable Shift Register/1
  freq/1 -> Register14/1
  Constant7/1 -> Subsystem1/1(Chan)
  Constant8/1 -> Subsystem2/1(Chan)
  Constant6/1 -> Subsystem/1(Chan)
  Register15/1 -> Subsystem1/3(In3), Subsystem2/3(In3), Subsystem/3(In3)
  "DDS Compiler 6.0 "/4 -> Register16/1
  "DDS Compiler 6.0 "/3 -> Register15/1
  "DDS Compiler 6.0 "/2 -> Register2/1
  Constant5/1 -> "DDS Compiler 6.0 "/3
  Constant4/1 -> "DDS Compiler 6.0 "/5
  Mux5/1 -> "DDS Compiler 6.0 "/2
  AddSub/1 -> Mux5/4
  Shift/1 -> Mux5/3, AddSub/2
  Register14/1 -> Mux5/2, AddSub/1, Shift/1
  Register13/1 -> "DDS Compiler 6.0 "/1
  Constant3/1 -> Addressable Shift Register1/2
  Register12/1 -> Assert1/1, Mux5/1, Register1/1
  Addressable Shift Register1/1 -> Register12/1
  Constant/1 -> Addressable Shift Register/2
  Register8/1 -> Assert/1, Register13/1
  Addressable Shift Register/1 -> Register8/1
  "DDS Compiler 6.0 "/6 -> Terminator1/1
  "DDS Compiler 6.0 "/1 -> Terminator/1
  "DDS Compiler 6.0 "/7 -> Terminator2/1

== system CryoDetHcd/DspCore/DSP/channel_processor/channel_processor_x4/128_channel_processor4/Variant Subsystem/LMS/controller/1st_harmonic ==
  note: D=16
  note: D=2
  note: D=5
  error : Inport
  gain : Inport  Port=2
  delay : Inport  Port=3
  enable : Inport  Port=4
  cos : Inport  Port=5
  sin : Inport  Port=6
  AddSub4 : xbsIndex_r4/AddSub  mode=Addition  use_carryin=off  use_carryout=off  en=off  latency=3  precision=User Defined  arith_type="Signed  (2's comp)"  n_bits=32  bin_pt=31  quantization=Truncate  overflow=Wrap  use_behavioral_HDL=off  hw_selection=Fabric  pipelined=off  dbl_ovrd=off  block_type=addsub
  Addressable Shift Register : xbsIndex_r4/Addressable Shift Register  infer_latency=off  depth=8  initVector=[0]  en=off  use_behavioral_HDL=off  Optimization=Resource  dbl_ovrd=off  block_type=addrsr
      settings: infoedit="Delay of configurable length.  Any element in the delay line can be addressed and driven onto the output port.<br><br>Hardware notes: Generates fast, compact FIFO-style shift registers or delay lines using SRL16/SRL32 mode of the slice LUTs"
  Addressable Shift Register1 : xbsIndex_r4/Addressable Shift Register  infer_latency=off  depth=8  initVector=[0]  en=off  use_behavioral_HDL=off  Optimization=Resource  dbl_ovrd=off  block_type=addrsr
      settings: infoedit="Delay of configurable length.  Any element in the delay line can be addressed and driven onto the output port.<br><br>Hardware notes: Generates fast, compact FIFO-style shift registers or delay lines using SRL16/SRL32 mode of the slice LUTs"
  Delay1 : xbsIndex_r4/Delay  rst=off  infoeditControl=Selection of Reset will increase slice count due to use of real FFs and instead of SRLs  en=off  latency=5  reg_retiming=off  dbl_ovrd=off  block_type=delay
  Down Sample1 : xbsIndex_r4/Down Sample  sample_ratio=128  sample_phase=First Value of Frame  en=off  rst=off  latency=0  dbl_ovrd=off  block_type=dsamp
  Down Sample2 : xbsIndex_r4/Down Sample  sample_ratio=128  sample_phase=First Value of Frame  en=off  rst=off  latency=0  dbl_ovrd=off  block_type=dsamp
  Down Sample3 : xbsIndex_r4/Down Sample  sample_ratio=128  sample_phase=First Value of Frame  en=off  rst=off  latency=0  dbl_ovrd=off  block_type=dsamp
  Mult{,1,7,13} (4 alike) : xbsIndex_r4/Mult  precision=User Defined  arith_type="Signed  (2's comp)"  n_bits=32  bin_pt=32  quantization=Truncate  overflow=Wrap  en=off  latency=3  use_behavioral_HDL=off  opt=Speed  use_embedded=on  optimum_pipeline=off  pipeline=on  dbl_ovrd=off  use_rpm=on  placement_style=Triangular  block_type=mult
  Subsystem : Subsystem
  Subsystem1 : Subsystem
  Up Sample : xbsIndex_r4/Up Sample  sample_ratio=128  copy_samples=on  en=off  latency=1  dbl_ovrd=off  block_type=usamp
  Up Sample1 : xbsIndex_r4/Up Sample  sample_ratio=128  copy_samples=on  en=off  latency=1  dbl_ovrd=off  block_type=usamp
  interleaved_accumulator1 : Subsystem
  interleaved_accumulator2 : Subsystem
  alpha1 : Outport
  alpha2 : Outport  Port=2
  Out3 : Outport  Port=3
  wires:
  error/1 -> Mult13/1, Mult7/1
  sin/1 -> Down Sample1/1, Mult/2
  cos/1 -> Down Sample2/1, Mult1/2
  Mult7/1 -> Subsystem1/2(in)
  Mult13/1 -> Subsystem/2(in)
  Mult/1 -> AddSub4/1
  Mult1/1 -> AddSub4/2
  AddSub4/1 -> Out3/1
  interleaved_accumulator2/1(Out1) -> alpha2/1, Mult1/1  "alpha2"
  interleaved_accumulator1/1(Out1) -> alpha1/1, Mult/1  "alpha1"
  Subsystem/1(out) -> interleaved_accumulator1/1(In1)
  Down Sample1/1 -> Addressable Shift Register/1
  Down Sample2/1 -> Addressable Shift Register1/1
  Addressable Shift Register1/1 -> Up Sample/1
  Addressable Shift Register/1 -> Up Sample1/1
  delay/1 -> Down Sample3/1
  Subsystem1/1(out) -> interleaved_accumulator2/1(In1)
  gain/1 -> Subsystem1/1(gain), Subsystem/1(gain)
  Down Sample3/1 -> Addressable Shift Register1/2, Addressable Shift Register/2
  Up Sample/1 -> Mult7/2
  Up Sample1/1 -> Mult13/2
  enable/1 -> Delay1/1
  Delay1/1 -> interleaved_accumulator2/2(enable), interleaved_accumulator1/2(enable)

== system CryoDetHcd/DspCore/DSP/channel_processor/channel_processor_x4/128_channel_processor4/Variant Subsystem/LMS/controller/1st_harmonic1 ==
  note: D=5
  note: D=2
  note: D=16
  error : Inport
  gain : Inport  Port=2
  delay : Inport  Port=3
  enable : Inport  Port=4
  cos : Inport  Port=5
  sin : Inport  Port=6
  AddSub4 : xbsIndex_r4/AddSub  mode=Addition  use_carryin=off  use_carryout=off  en=off  latency=3  precision=User Defined  arith_type="Signed  (2's comp)"  n_bits=32  bin_pt=31  quantization=Truncate  overflow=Wrap  use_behavioral_HDL=off  hw_selection=Fabric  pipelined=off  dbl_ovrd=off  block_type=addsub
  Addressable Shift Register : xbsIndex_r4/Addressable Shift Register  infer_latency=off  depth=8  initVector=[0]  en=off  use_behavioral_HDL=off  Optimization=Resource  dbl_ovrd=off  block_type=addrsr
      settings: infoedit="Delay of configurable length.  Any element in the delay line can be addressed and driven onto the output port.<br><br>Hardware notes: Generates fast, compact FIFO-style shift registers or delay lines using SRL16/SRL32 mode of the slice LUTs"
  Addressable Shift Register1 : xbsIndex_r4/Addressable Shift Register  infer_latency=off  depth=8  initVector=[0]  en=off  use_behavioral_HDL=off  Optimization=Resource  dbl_ovrd=off  block_type=addrsr
      settings: infoedit="Delay of configurable length.  Any element in the delay line can be addressed and driven onto the output port.<br><br>Hardware notes: Generates fast, compact FIFO-style shift registers or delay lines using SRL16/SRL32 mode of the slice LUTs"
  Delay1 : xbsIndex_r4/Delay  rst=off  infoeditControl=Selection of Reset will increase slice count due to use of real FFs and instead of SRLs  en=off  latency=5  reg_retiming=off  dbl_ovrd=off  block_type=delay
  Down Sample1 : xbsIndex_r4/Down Sample  sample_ratio=128  sample_phase=First Value of Frame  en=off  rst=off  latency=0  dbl_ovrd=off  block_type=dsamp
  Down Sample2 : xbsIndex_r4/Down Sample  sample_ratio=128  sample_phase=First Value of Frame  en=off  rst=off  latency=0  dbl_ovrd=off  block_type=dsamp
  Down Sample3 : xbsIndex_r4/Down Sample  sample_ratio=128  sample_phase=First Value of Frame  en=off  rst=off  latency=0  dbl_ovrd=off  block_type=dsamp
  Mult{,1,7,13} (4 alike) : xbsIndex_r4/Mult  precision=User Defined  arith_type="Signed  (2's comp)"  n_bits=32  bin_pt=32  quantization=Truncate  overflow=Wrap  en=off  latency=3  use_behavioral_HDL=off  opt=Speed  use_embedded=on  optimum_pipeline=off  pipeline=on  dbl_ovrd=off  use_rpm=on  placement_style=Triangular  block_type=mult
  Subsystem : Subsystem
  Subsystem1 : Subsystem
  Up Sample : xbsIndex_r4/Up Sample  sample_ratio=128  copy_samples=on  en=off  latency=1  dbl_ovrd=off  block_type=usamp
  Up Sample1 : xbsIndex_r4/Up Sample  sample_ratio=128  copy_samples=on  en=off  latency=1  dbl_ovrd=off  block_type=usamp
  interleaved_accumulator1 : Subsystem
  interleaved_accumulator2 : Subsystem
  alpha1 : Outport
  alpha2 : Outport  Port=2
  Out3 : Outport  Port=3
  wires:
  Delay1/1 -> interleaved_accumulator1/2(enable), interleaved_accumulator2/2(enable)
  enable/1 -> Delay1/1
  Up Sample1/1 -> Mult13/2
  Up Sample/1 -> Mult7/2
  Down Sample3/1 -> Addressable Shift Register/2, Addressable Shift Register1/2
  gain/1 -> Subsystem/1(gain), Subsystem1/1(gain)
  Subsystem1/1(out) -> interleaved_accumulator2/1(In1)
  delay/1 -> Down Sample3/1
  Addressable Shift Register/1 -> Up Sample1/1
  Addressable Shift Register1/1 -> Up Sample/1
  Down Sample2/1 -> Addressable Shift Register1/1
  Down Sample1/1 -> Addressable Shift Register/1
  Subsystem/1(out) -> interleaved_accumulator1/1(In1)
  interleaved_accumulator1/1(Out1) -> Mult/1, alpha1/1  "alpha1"
  interleaved_accumulator2/1(Out1) -> Mult1/1, alpha2/1  "alpha2"
  AddSub4/1 -> Out3/1
  Mult1/1 -> AddSub4/2
  Mult/1 -> AddSub4/1
  Mult13/1 -> Subsystem/2(in)
  Mult7/1 -> Subsystem1/2(in)
  cos/1 -> Mult1/2, Down Sample2/1
  sin/1 -> Mult/2, Down Sample1/1
  error/1 -> Mult7/1, Mult13/1
